simulink model "Test_FourMotor_PID_Ave"  (R2025a)
settings: Solver=ode4  StartTime=0.0  StopTime=2  FixedStep=60e-6  RelTol=1e-3
values from neighbouring files (symbols this model uses):
  Ts = 2e-6    (= 2e-06)    [param.m]
  ts_vec = 60e-6    (= 6e-05)    [param.m]
undefined symbols (not defined in the file or in its folder): DiscIntNeverNeededParam, gcbh, HEV_Param, Limit, magnitude, motorctrl, RPM, sps_rtmsupport
libraries: fl_lib x39, spsCurrentMeasurementLib x26, spsIdealSwitchLib x24, nesl_utility x22, spsVoltageMeasurementLib x21, simulink_extras x13, spsControlledCurrentSourceLib x12, spsControlledVoltageSourceLib x9, slpidlib x7, simulink x6, Uav_Electrical_lib x5, spsSeriesRLCBranchLib x4
(part 1 of 5)
settings Model: Creator=froshoo  LastModifiedBy=froshoo
settings DataIOCC: SaveOutput=off  SignalLogging=off  DSMLogging=off  SaveTime=off  ReturnWorkspaceOutputs=off
settings SimscapeCC: SimscapeLogType=all  SimscapeLogSimulationStatistics=on  SimscapeLogToSDI=on  SimscapeLogOpenViewer=on

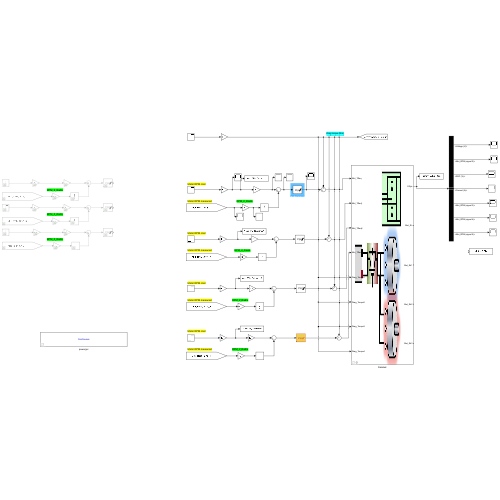
[thumbnail: Simulink's stored preview of the top-level diagram]
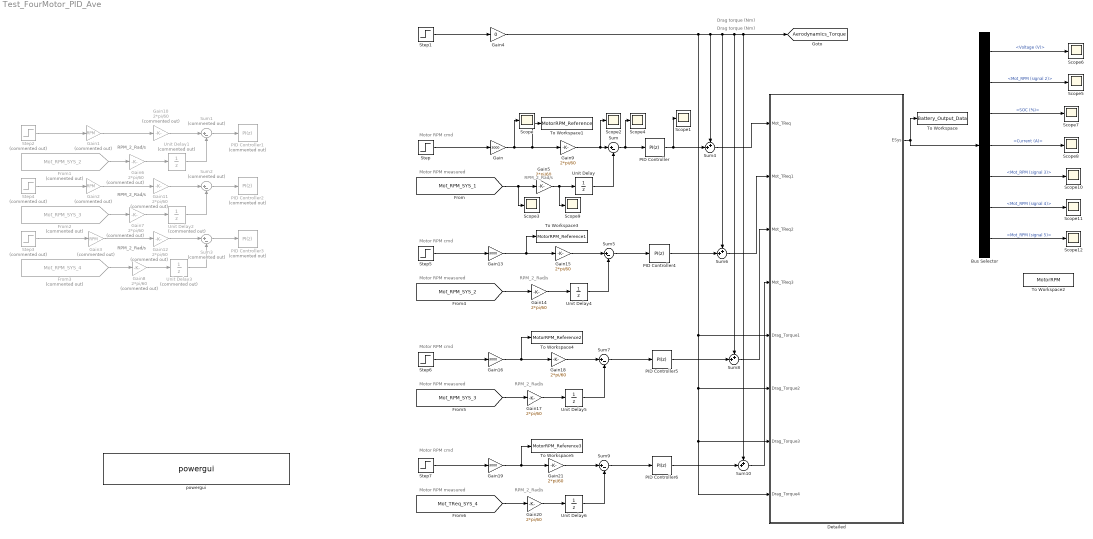
== system Test_FourMotor_PID_Ave ==
  note: Motor RPM cmd
  note: Motor RPM measured
  note: RPM_2_Rad/s
  note: RPM_2_Rad/s
  note: RPM_2_Rad/s
  note: RPM_2_Rad/s
  note: Drag torque (Nm)
  note: Drag torque (Nm)
  note: RPM_2_Rad/s
  note: Motor RPM cmd
  note: Motor RPM measured
  note: Motor RPM measured
  note: RPM_2_Rad/s
  note: Motor RPM cmd
  note: Motor RPM cmd
  note: Motor RPM measured
  note: RPM_2_Rad/s
  Bus Selector : BusSelector  OutputSignals=Batt (signal 1).Voltage (V),Mot_RPM (signal 2),Batt (signal 1).SOC (%),Batt (signal 1).Current (A),Mot_RPM (signal 3),Mot_RPM (signal 4),Mot_RPM (signal 5)
  Detailed : Subsystem  AncestorBlock=Uav_Electrical_lib/Detailed  mask{popup_batteryvariant=Cells}
      mask prompts: popup_batteryvariant "Battery Model"
      mask init:
      | set_param([gcb '/Battery'],'LabelModeActiveChoice',get_param(gcb,'popup_batteryvariant'));
      mask TypeOptions popup_batteryvariant: Predefined | Cells | Generic
      mask Display: image('HEV_Electrical_Detailed_IMAGE.jpg');
  From1 : From  Commented=on  GotoTag=Mot_RPM_SYS_2  TagVisibility=global
  From2 : From  Commented=on  GotoTag=Mot_RPM_SYS_3  TagVisibility=global
  From3 : From  Commented=on  GotoTag=Mot_RPM_SYS_4  TagVisibility=global
  Gain{,13,16,19} (4 alike) : Gain  Gain=3000
  Gain1 : Gain  Commented=on  Gain=RPM
  Gain{6..8,10..12} (6 alike) : Gain  Commented=on  Gain=2*pi/60
  Gain{5,9,14..15,17..18,20..21} (8 alike) : Gain  Gain=2*pi/60
  Gain2 : Gain  Commented=on  Gain=RPM
  Gain3 : Gain  Commented=on  Gain=RPM
  Gain4 : Gain  Gain=0
  PID Controller{,4..6} (4 alike) : slpidlib/PID Controller  Controller=PI  Form=Parallel  TimeDomain=Discrete-time  UseExternalTs=off  SampleTime=0.005  IntegratorMethod=Forward Euler  FilterMethod=Forward Euler  ControllerParametersSource=internal  P=0.4  I=0.5  UseKiTs=off  D=motorctrl.d  UseExternalDerivativeSource=off  N=motorctrl.n  UseFilter=on  TunerSelectOption=Transfer Function Based (PID Tuner App)  InitialConditionSource=internal  InitialConditionForIntegrator=0  InitialConditionForFilter=0  DifferentiatorICPrevScaledInput=0  ExternalReset=none  TrackingMode=off  Kt=1  LimitOutput=on  SatLimitsSource=internal  UpperSaturationLimit=800  LowerSaturationLimit=-800  LinearizeAsGain=on  AntiWindupMode=back-calculation  Kb=1  LimitIntegrator=off  UpperIntegratorSaturationLimit=inf  LowerIntegratorSaturationLimit=-inf  POutMin=[]  POutMax=[]  IOutMin=[]  IOutMax=[]  DOutMin=[]  DOutMax=[]  NOutMin=[]  NOutMax=[]  SumOutMin=[]  SumOutMax=[]  SaturationOutMin=[]  SaturationOutMax=[]  PParamMin=[]  PParamMax=[]  IParamMin=[]  IParamMax=[]  DParamMin=[]  DParamMax=[]  NParamMin=[]  NParamMax=[]  KbParamMin=[]  KbParamMax=[]  KtParamMin=[]  KtParamMax=[]  KbOutMin=[]  KbOutMax=[]  KtOutMin=[]  KtOutMax=[]  IntegratorOutMin=[]  IntegratorOutMax=[]  FilterOutMin=[]  FilterOutMax=[]  SumI1OutMin=[]  SumI1OutMax=[]  SumI2OutMin=[]  SumI2OutMax=[]  SumI3OutMin=[]  SumI3OutMax=[]  SumI4OutMin=[]  SumI4OutMax=[]  SumDOutMin=[]  SumDOutMax=[]  DifferentiatorOutMin=[]  DifferentiatorOutMax=[]  FilterDiffOutCoefMin=[]  FilterDiffOutCoefMax=[]  ReciprocalOutMin=[]  ReciprocalOutMax=[]  SumDenOutMin=[]  SumDenOutMax=[]  SumNumOutMin=[]  SumNumOutMax=[]  DivideOutMin=[]  DivideOutMax=[]  UdiffTsProdOutMin=[]  UdiffTsProdOutMax=[]  NTsProdOutMin=[]  NTsProdOutMax=[]  UintegralTsProdOutMin=[]  UintegralTsProdOutMax=[]  UngainTsProdOutMin=[]  UngainTsProdOutMax=[]  ClampingZeroOutDataTypeStr=Inherit: Inherit via back propagation  ClampingZeroOutMin=[]  ClampingZeroOutMax=[]  FilterDenConstantOutDataTypeStr=Inherit: Inherit via back propagation  FilterDenConstantOutMin=[]  FilterDenConstantOutMax=[]  PCopyOutDataTypeStr=Inherit: Inherit via back propagation  PCopyOutMin=[]  PCopyOutMax=[]  NCopyOutDataTypeStr=Inherit: Inherit via back propagation  NCopyOutMin=[]  NCopyOutMax=[]  IntegratorContinuousStateAttributes=''  IntegratorStateMustResolveToSignalObject=off  IntegratorRTWStateStorageClass=Auto  FilterContinuousStateAttributes=''  FilterStateMustResolveToSignalObject=off  FilterRTWStateStorageClass=Auto  ParallelPVariant=InternalParameters  IdealPVariant=Disabled  IVariant=InternalParameters  DVariant=Disabled  IntegratorVariant=Discrete  SatVariant=Enabled  AWVariant=BackCalculation  PCopyVariant=Disabled  TRVariant=Disabled  FdbkBlocksVariant=Forward  IdealPFdbkVariant=Disabled  SatFdbkVariant=Disabled  DerivativeFilterVariant=Disabled  NVariant=Disabled  NCopyVariant=Disabled_SignalSpec  FilterICVariant=Disabled  IntegratorICVariant=InternalICs  ExternalResetVariant=Disabled  TRSumVariant=Passthrough  SumFdbkVariant=Disabled  SumVariant=Sum_PI  TsampFilterVariant=InternalTs  TsampNgainVariant=Passthrough  TsampIntegralVariant=Disabled_SignalSpec  ExternalSaturationOutDataTypeStr=Inherit: Same as second input  DerivativeSourceVariant=Disabled  PreIntVariant=InternalPreInt
  PID Controller1 : slpidlib/PID Controller  Commented=on  Controller=PI  Form=Parallel  TimeDomain=Discrete-time  UseExternalTs=off  SampleTime=0.005  IntegratorMethod=Forward Euler  FilterMethod=Forward Euler  ControllerParametersSource=internal  P=motorctrl.p  I=motorctrl.i  UseKiTs=off  D=motorctrl.d  UseExternalDerivativeSource=off  N=motorctrl.n  UseFilter=on  TunerSelectOption=Transfer Function Based (PID Tuner App)  InitialConditionSource=internal  InitialConditionForIntegrator=0  InitialConditionForFilter=0  DifferentiatorICPrevScaledInput=0  ExternalReset=none  TrackingMode=off  Kt=1  LimitOutput=on  SatLimitsSource=internal  UpperSaturationLimit=Limit  LowerSaturationLimit=-Limit  LinearizeAsGain=on  AntiWindupMode=back-calculation  Kb=1  LimitIntegrator=off  UpperIntegratorSaturationLimit=inf  LowerIntegratorSaturationLimit=-inf  POutMin=[]  POutMax=[]  IOutMin=[]  IOutMax=[]  DOutMin=[]  DOutMax=[]  NOutMin=[]  NOutMax=[]  SumOutMin=[]  SumOutMax=[]  SaturationOutMin=[]  SaturationOutMax=[]  PParamMin=[]  PParamMax=[]  IParamMin=[]  IParamMax=[]  DParamMin=[]  DParamMax=[]  NParamMin=[]  NParamMax=[]  KbParamMin=[]  KbParamMax=[]  KtParamMin=[]  KtParamMax=[]  KbOutMin=[]  KbOutMax=[]  KtOutMin=[]  KtOutMax=[]  IntegratorOutMin=[]  IntegratorOutMax=[]  FilterOutMin=[]  FilterOutMax=[]  SumI1OutMin=[]  SumI1OutMax=[]  SumI2OutMin=[]  SumI2OutMax=[]  SumI3OutMin=[]  SumI3OutMax=[]  SumI4OutMin=[]  SumI4OutMax=[]  SumDOutMin=[]  SumDOutMax=[]  DifferentiatorOutMin=[]  DifferentiatorOutMax=[]  FilterDiffOutCoefMin=[]  FilterDiffOutCoefMax=[]  ReciprocalOutMin=[]  ReciprocalOutMax=[]  SumDenOutMin=[]  SumDenOutMax=[]  SumNumOutMin=[]  SumNumOutMax=[]  DivideOutMin=[]  DivideOutMax=[]  UdiffTsProdOutMin=[]  UdiffTsProdOutMax=[]  NTsProdOutMin=[]  NTsProdOutMax=[]  UintegralTsProdOutMin=[]  UintegralTsProdOutMax=[]  UngainTsProdOutMin=[]  UngainTsProdOutMax=[]  ClampingZeroOutDataTypeStr=Inherit: Inherit via back propagation  ClampingZeroOutMin=[]  ClampingZeroOutMax=[]  FilterDenConstantOutDataTypeStr=Inherit: Inherit via back propagation  FilterDenConstantOutMin=[]  FilterDenConstantOutMax=[]  PCopyOutDataTypeStr=Inherit: Inherit via back propagation  PCopyOutMin=[]  PCopyOutMax=[]  NCopyOutDataTypeStr=Inherit: Inherit via back propagation  NCopyOutMin=[]  NCopyOutMax=[]  IntegratorContinuousStateAttributes=''  IntegratorStateMustResolveToSignalObject=off  IntegratorRTWStateStorageClass=Auto  FilterContinuousStateAttributes=''  FilterStateMustResolveToSignalObject=off  FilterRTWStateStorageClass=Auto  ParallelPVariant=InternalParameters  IdealPVariant=Disabled  IVariant=InternalParameters  DVariant=Disabled  IntegratorVariant=Discrete  SatVariant=Enabled  AWVariant=BackCalculation  PCopyVariant=Disabled  TRVariant=Disabled  FdbkBlocksVariant=Forward  IdealPFdbkVariant=Disabled  SatFdbkVariant=Disabled  DerivativeFilterVariant=Disabled  NVariant=Disabled  NCopyVariant=Disabled_SignalSpec  FilterICVariant=Disabled  IntegratorICVariant=InternalICs  ExternalResetVariant=Disabled  TRSumVariant=Passthrough  SumFdbkVariant=Disabled  SumVariant=Sum_PI  TsampFilterVariant=InternalTs  TsampNgainVariant=Passthrough  TsampIntegralVariant=Disabled_SignalSpec  ExternalSaturationOutDataTypeStr=Inherit: Same as second input  DerivativeSourceVariant=Disabled  PreIntVariant=InternalPreInt
  PID Controller2 : slpidlib/PID Controller  Commented=on  Controller=PI  Form=Parallel  TimeDomain=Discrete-time  UseExternalTs=off  SampleTime=0.005  IntegratorMethod=Forward Euler  FilterMethod=Forward Euler  ControllerParametersSource=internal  P=motorctrl.p  I=motorctrl.i  UseKiTs=off  D=motorctrl.d  UseExternalDerivativeSource=off  N=motorctrl.n  UseFilter=on  TunerSelectOption=Transfer Function Based (PID Tuner App)  InitialConditionSource=internal  InitialConditionForIntegrator=0  InitialConditionForFilter=0  DifferentiatorICPrevScaledInput=0  ExternalReset=none  TrackingMode=off  Kt=1  LimitOutput=on  SatLimitsSource=internal  UpperSaturationLimit=Limit  LowerSaturationLimit=-Limit  LinearizeAsGain=on  AntiWindupMode=back-calculation  Kb=1  LimitIntegrator=off  UpperIntegratorSaturationLimit=inf  LowerIntegratorSaturationLimit=-inf  POutMin=[]  POutMax=[]  IOutMin=[]  IOutMax=[]  DOutMin=[]  DOutMax=[]  NOutMin=[]  NOutMax=[]  SumOutMin=[]  SumOutMax=[]  SaturationOutMin=[]  SaturationOutMax=[]  PParamMin=[]  PParamMax=[]  IParamMin=[]  IParamMax=[]  DParamMin=[]  DParamMax=[]  NParamMin=[]  NParamMax=[]  KbParamMin=[]  KbParamMax=[]  KtParamMin=[]  KtParamMax=[]  KbOutMin=[]  KbOutMax=[]  KtOutMin=[]  KtOutMax=[]  IntegratorOutMin=[]  IntegratorOutMax=[]  FilterOutMin=[]  FilterOutMax=[]  SumI1OutMin=[]  SumI1OutMax=[]  SumI2OutMin=[]  SumI2OutMax=[]  SumI3OutMin=[]  SumI3OutMax=[]  SumI4OutMin=[]  SumI4OutMax=[]  SumDOutMin=[]  SumDOutMax=[]  DifferentiatorOutMin=[]  DifferentiatorOutMax=[]  FilterDiffOutCoefMin=[]  FilterDiffOutCoefMax=[]  ReciprocalOutMin=[]  ReciprocalOutMax=[]  SumDenOutMin=[]  SumDenOutMax=[]  SumNumOutMin=[]  SumNumOutMax=[]  DivideOutMin=[]  DivideOutMax=[]  UdiffTsProdOutMin=[]  UdiffTsProdOutMax=[]  NTsProdOutMin=[]  NTsProdOutMax=[]  UintegralTsProdOutMin=[]  UintegralTsProdOutMax=[]  UngainTsProdOutMin=[]  UngainTsProdOutMax=[]  ClampingZeroOutDataTypeStr=Inherit: Inherit via back propagation  ClampingZeroOutMin=[]  ClampingZeroOutMax=[]  FilterDenConstantOutDataTypeStr=Inherit: Inherit via back propagation  FilterDenConstantOutMin=[]  FilterDenConstantOutMax=[]  PCopyOutDataTypeStr=Inherit: Inherit via back propagation  PCopyOutMin=[]  PCopyOutMax=[]  NCopyOutDataTypeStr=Inherit: Inherit via back propagation  NCopyOutMin=[]  NCopyOutMax=[]  IntegratorContinuousStateAttributes=''  IntegratorStateMustResolveToSignalObject=off  IntegratorRTWStateStorageClass=Auto  FilterContinuousStateAttributes=''  FilterStateMustResolveToSignalObject=off  FilterRTWStateStorageClass=Auto  ParallelPVariant=InternalParameters  IdealPVariant=Disabled  IVariant=InternalParameters  DVariant=Disabled  IntegratorVariant=Discrete  SatVariant=Enabled  AWVariant=BackCalculation  PCopyVariant=Disabled  TRVariant=Disabled  FdbkBlocksVariant=Forward  IdealPFdbkVariant=Disabled  SatFdbkVariant=Disabled  DerivativeFilterVariant=Disabled  NVariant=Disabled  NCopyVariant=Disabled_SignalSpec  FilterICVariant=Disabled  IntegratorICVariant=InternalICs  ExternalResetVariant=Disabled  TRSumVariant=Passthrough  SumFdbkVariant=Disabled  SumVariant=Sum_PI  TsampFilterVariant=InternalTs  TsampNgainVariant=Passthrough  TsampIntegralVariant=Disabled_SignalSpec  ExternalSaturationOutDataTypeStr=Inherit: Same as second input  DerivativeSourceVariant=Disabled  PreIntVariant=InternalPreInt
  PID Controller3 : slpidlib/PID Controller  Commented=on  Controller=PI  Form=Parallel  TimeDomain=Discrete-time  UseExternalTs=off  SampleTime=0.005  IntegratorMethod=Forward Euler  FilterMethod=Forward Euler  ControllerParametersSource=internal  P=motorctrl.p  I=motorctrl.i  UseKiTs=off  D=motorctrl.d  UseExternalDerivativeSource=off  N=motorctrl.n  UseFilter=on  TunerSelectOption=Transfer Function Based (PID Tuner App)  InitialConditionSource=internal  InitialConditionForIntegrator=0  InitialConditionForFilter=0  DifferentiatorICPrevScaledInput=0  ExternalReset=none  TrackingMode=off  Kt=1  LimitOutput=on  SatLimitsSource=internal  UpperSaturationLimit=Limit  LowerSaturationLimit=-Limit  LinearizeAsGain=on  AntiWindupMode=back-calculation  Kb=1  LimitIntegrator=off  UpperIntegratorSaturationLimit=inf  LowerIntegratorSaturationLimit=-inf  POutMin=[]  POutMax=[]  IOutMin=[]  IOutMax=[]  DOutMin=[]  DOutMax=[]  NOutMin=[]  NOutMax=[]  SumOutMin=[]  SumOutMax=[]  SaturationOutMin=[]  SaturationOutMax=[]  PParamMin=[]  PParamMax=[]  IParamMin=[]  IParamMax=[]  DParamMin=[]  DParamMax=[]  NParamMin=[]  NParamMax=[]  KbParamMin=[]  KbParamMax=[]  KtParamMin=[]  KtParamMax=[]  KbOutMin=[]  KbOutMax=[]  KtOutMin=[]  KtOutMax=[]  IntegratorOutMin=[]  IntegratorOutMax=[]  FilterOutMin=[]  FilterOutMax=[]  SumI1OutMin=[]  SumI1OutMax=[]  SumI2OutMin=[]  SumI2OutMax=[]  SumI3OutMin=[]  SumI3OutMax=[]  SumI4OutMin=[]  SumI4OutMax=[]  SumDOutMin=[]  SumDOutMax=[]  DifferentiatorOutMin=[]  DifferentiatorOutMax=[]  FilterDiffOutCoefMin=[]  FilterDiffOutCoefMax=[]  ReciprocalOutMin=[]  ReciprocalOutMax=[]  SumDenOutMin=[]  SumDenOutMax=[]  SumNumOutMin=[]  SumNumOutMax=[]  DivideOutMin=[]  DivideOutMax=[]  UdiffTsProdOutMin=[]  UdiffTsProdOutMax=[]  NTsProdOutMin=[]  NTsProdOutMax=[]  UintegralTsProdOutMin=[]  UintegralTsProdOutMax=[]  UngainTsProdOutMin=[]  UngainTsProdOutMax=[]  ClampingZeroOutDataTypeStr=Inherit: Inherit via back propagation  ClampingZeroOutMin=[]  ClampingZeroOutMax=[]  FilterDenConstantOutDataTypeStr=Inherit: Inherit via back propagation  FilterDenConstantOutMin=[]  FilterDenConstantOutMax=[]  PCopyOutDataTypeStr=Inherit: Inherit via back propagation  PCopyOutMin=[]  PCopyOutMax=[]  NCopyOutDataTypeStr=Inherit: Inherit via back propagation  NCopyOutMin=[]  NCopyOutMax=[]  IntegratorContinuousStateAttributes=''  IntegratorStateMustResolveToSignalObject=off  IntegratorRTWStateStorageClass=Auto  FilterContinuousStateAttributes=''  FilterStateMustResolveToSignalObject=off  FilterRTWStateStorageClass=Auto  ParallelPVariant=InternalParameters  IdealPVariant=Disabled  IVariant=InternalParameters  DVariant=Disabled  IntegratorVariant=Discrete  SatVariant=Enabled  AWVariant=BackCalculation  PCopyVariant=Disabled  TRVariant=Disabled  FdbkBlocksVariant=Forward  IdealPFdbkVariant=Disabled  SatFdbkVariant=Disabled  DerivativeFilterVariant=Disabled  NVariant=Disabled  NCopyVariant=Disabled_SignalSpec  FilterICVariant=Disabled  IntegratorICVariant=InternalICs  ExternalResetVariant=Disabled  TRSumVariant=Passthrough  SumFdbkVariant=Disabled  SumVariant=Sum_PI  TsampFilterVariant=InternalTs  TsampNgainVariant=Passthrough  TsampIntegralVariant=Disabled_SignalSpec  ExternalSaturationOutDataTypeStr=Inherit: Same as second input  DerivativeSourceVariant=Disabled  PreIntVariant=InternalPreInt
  Scope{,1..12} (13 alike) : Scope
      Scope settings: ActiveDisplayYMinimum=2000  ActiveDisplayYMaximum=4000
      Scope1 settings: ActiveDisplayYMinimum=-481.89960137193771  ActiveDisplayYMaximum=332.79708047153025
      Scope10 settings: ActiveDisplayYMinimum=-838.99189969639019  ActiveDisplayYMaximum=7550.927097267514  DataLoggingVariableName=ScopeData18
      Scope11 settings: ActiveDisplayYMinimum=-838.99189969639019  ActiveDisplayYMaximum=7550.927097267514  DataLoggingVariableName=ScopeData22
      Scope12 settings: ActiveDisplayYMinimum=-838.99189969639019  ActiveDisplayYMaximum=7550.927097267514  DataLoggingVariableName=ScopeData23
      Scope2 settings: ActiveDisplayYMinimum=214.15926535897933  ActiveDisplayYMaximum=414.15926535897933  DataLoggingVariableName=ScopeData17
      Scope3 settings: ActiveDisplayYMinimum=-1  ActiveDisplayYMaximum=1  DataLoggingVariableName=ScopeData19
      Scope4 settings: ActiveDisplayYMinimum=-39.421537573321494  ActiveDisplayYMaximum=353.44602124034606  DataLoggingVariableName=ScopeData20
      Scope5 settings: ActiveDisplayYMinimum=-838.99189969639019  ActiveDisplayYMaximum=7550.927097267514  DataLoggingVariableName=ScopeData2
      Scope6 settings: ActiveDisplayYMinimum=813.40102643578655  ActiveDisplayYMaximum=813.74696487540177  DataLoggingVariableName=ScopeData3
      Scope7 settings: ActiveDisplayYMinimum=99.00226  ActiveDisplayYMaximum=100.11086  DataLoggingVariableName=ScopeData4
      Scope8 settings: ActiveDisplayYMinimum=-1508.9225284750978  ActiveDisplayYMaximum=1817.2458957057474  DataLoggingVariableName=ScopeData5
      Scope9 settings: ActiveDisplayYMinimum=-39.286755881366751  ActiveDisplayYMaximum=353.5808029323008  DataLoggingVariableName=ScopeData21
  Step{,1,5..7} (5 alike) : Step  Time=0  SampleTime=0
  Step2 : Step  Commented=on  Time=0  SampleTime=0
  Step3 : Step  Commented=on  Time=0  SampleTime=0
  Step4 : Step  Commented=on  Time=0  SampleTime=0
  Sum{,5,7,9} (4 alike) : Sum  Inputs=|+-
  Sum1 : Sum  Commented=on  Inputs=|+-
  Sum{4,6,8,10} (4 alike) : Sum  Inputs=++|
  Sum2 : Sum  Commented=on  Inputs=|+-
  Sum3 : Sum  Commented=on  Inputs=|+-
  To Workspace : ToWorkspace  VariableName=Battery_Output_Data  SaveFormat=Timeseries  SampleTime=-1
  To Workspace1 : ToWorkspace  VariableName=MotorRPM_Reference  SaveFormat=Timeseries  SampleTime=-1
  To Workspace2 : ToWorkspace  VariableName=MotorRPM  SaveFormat=Timeseries  SampleTime=-1
  To Workspace3 : ToWorkspace  VariableName=MotorRPM_Reference1  SaveFormat=Timeseries  SampleTime=-1
  To Workspace4 : ToWorkspace  VariableName=MotorRPM_Reference2  SaveFormat=Timeseries  SampleTime=-1
  To Workspace5 : ToWorkspace  VariableName=MotorRPM_Reference3  SaveFormat=Timeseries  SampleTime=-1
  Unit Delay{,4..6} (4 alike) : UnitDelay  SampleTime=-1  HasFrameUpgradeWarning=on
  Unit Delay1 : UnitDelay  Commented=on  SampleTime=-1  HasFrameUpgradeWarning=on
  Unit Delay2 : UnitDelay  Commented=on  SampleTime=-1  HasFrameUpgradeWarning=on
  Unit Delay3 : UnitDelay  Commented=on  SampleTime=-1  HasFrameUpgradeWarning=on
  powergui : sps_lib/powergui  Priority=1  SimulationMode=Continuous  SampleTime=50e-6  frequency=60  Iterations=50  frequencyindice=0  Pbase=100e6  ErrMax=1e-4  UnitsV=kV  UnitsW=MW  buscounter=0  FunctionMessages=off  echomessages=off  EnableUseOfTLC=off  CurrentSourceSwitches=off  DisableSnubberDevices=off  DisableRonSwitches=off  DisableVfSwitches=off  DisplayEquations=off  AutomaticDiscreteSolvers=off  SolverType=Tustin/Backward Euler (TBE)  Interpol=off  ExternalGateDelay=off  methode=off  Ts=100  x0status=blocks  SPID=on  SwTol=0  HookPort=off  NonlinearTolerance=1e-4  nMaxIteration=100  ContinueOnMaxIteration=off  RestoreLinks=warning  ResistiveCurrentMeasurement=off  Frange=[0:2:500]  Ylog=off  Xlog=on  ShowGrid=off  save=off  variable=ZData  structure=0  ZoomFFT=off  StartTime=0.0  cycles=1  DisplayStyle=1  fundamental=60  FreqAxis=off  MaxFrequency=1000  frequencyindicesteady=1  RmsSteady=1  display=off
  tag scope: Aerodynamics_Torque=global
  wires:
  Sum/1 -> Scope4/1, PID Controller/1
  From1/1 -> Gain6/1
  Sum1/1 -> PID Controller1/1
  Sum2/1 -> PID Controller2/1
  From3/1 -> Gain8/1
  Sum3/1 -> PID Controller3/1
  Detailed/1(ESys) -> To Workspace/1, Bus Selector/1
  Step/1 -> Gain/1
  Step3/1 -> Gain3/1
  Step4/1 -> Gain2/1
  Step2/1 -> Gain1/1
  Gain/1 -> To Workspace1/1, Gain9/1, Scope/1
  Gain1/1 -> Gain10/1
  Gain2/1 -> Gain11/1
  Gain3/1 -> Gain12/1
  [Mot_RPM_SYS_1] -> Gain5/1, Scope3/1
  Unit Delay/1 -> Sum/2
  Unit Delay1/1 -> Sum1/2
  Unit Delay2/1 -> Sum2/2
  Unit Delay3/1 -> Sum3/2
  From2/1 -> Gain7/1
  Step1/1 -> Gain4/1
  Gain5/1 -> Scope9/1, Unit Delay/1
  Gain6/1 -> Unit Delay1/1
  Gain7/1 -> Unit Delay2/1
  Gain8/1 -> Unit Delay3/1
  Gain9/1 -> Scope2/1, Sum/1
  Gain10/1 -> Sum1/1
  Gain11/1 -> Sum2/1
  Gain12/1 -> Sum3/1
  PID Controller/1 -> Sum4/2, Scope1/1
  Sum4/1 -> Detailed/1(Mot_TReq)
  PID Controller4/1 -> Sum6/2
  Gain15/1 -> Sum5/1
  Sum5/1 -> PID Controller4/1
  [Mot_RPM_SYS_2] -> Gain14/1
  Sum6/1 -> Detailed/2(Mot_TReq1)
  Step5/1 -> Gain13/1
  Gain14/1 -> Unit Delay4/1
  Unit Delay4/1 -> Sum5/2
  Gain13/1 -> To Workspace3/1, Gain15/1
  Sum7/1 -> PID Controller5/1
  Gain18/1 -> Sum7/1
  PID Controller5/1 -> Sum8/2
  Gain17/1 -> Unit Delay5/1
  Step6/1 -> Gain16/1
  Gain16/1 -> To Workspace4/1, Gain18/1
  Sum8/1 -> Detailed/3(Mot_TReq2)
  [Mot_RPM_SYS_3] -> Gain17/1
  Unit Delay5/1 -> Sum7/2
  Unit Delay6/1 -> Sum9/2
  Gain21/1 -> Sum9/1
  Sum10/1 -> Detailed/4(Mot_TReq3)
  Step7/1 -> Gain19/1
  PID Controller6/1 -> Sum10/2
  Sum9/1 -> PID Controller6/1
  Gain19/1 -> To Workspace5/1, Gain21/1
  Gain20/1 -> Unit Delay6/1
  [Mot_TReq_SYS_4] -> Gain20/1
  Gain4/1 -> Detailed/5(Drag_Torque1), Detailed/6(Drag_Torque2), Detailed/7(Drag_Torque3), Detailed/8(Drag_Torque4), [Aerodynamics_Torque], Sum10/1, Sum8/1, Sum6/1, Sum4/1
  Bus Selector/1 -> Scope6/1  "<Voltage (V)>"
  Bus Selector/2 -> Scope5/1  "<Mot_RPM (signal 2)>"
  Bus Selector/3 -> Scope7/1  "<SOC (%)>"
  Bus Selector/4 -> Scope8/1  "<Current (A)>"
  Bus Selector/5 -> Scope10/1  "<Mot_RPM (signal 3)>"
  Bus Selector/6 -> Scope11/1  "<Mot_RPM (signal 4)>"
  Bus Selector/7 -> Scope12/1  "<Mot_RPM (signal 5)>"

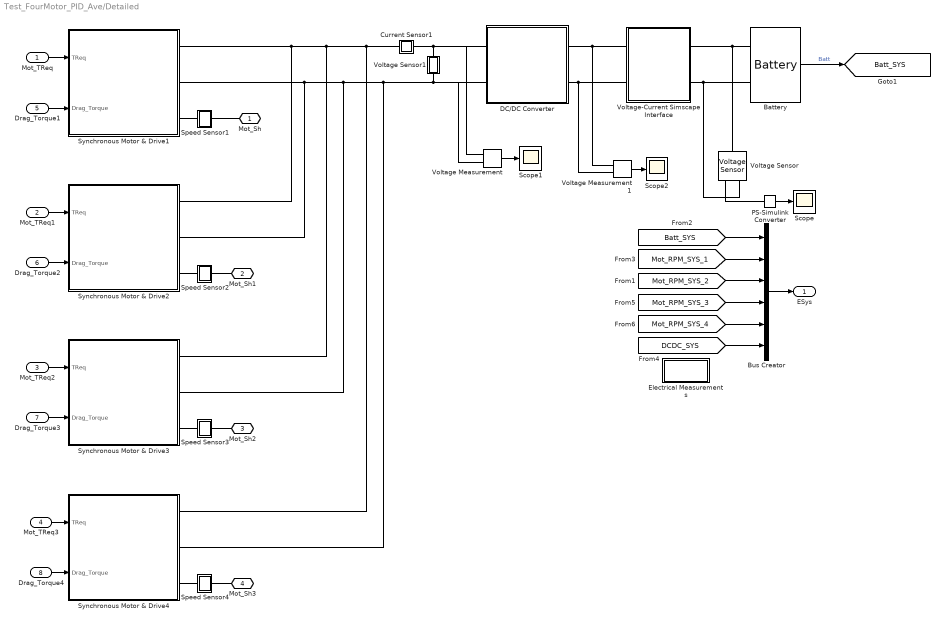
== system Test_FourMotor_PID_Ave/Detailed ==
  Mot_TReq : Inport
  Mot_TReq1 : Inport  Port=2
  Mot_TReq2 : Inport  Port=3
  Mot_TReq3 : Inport  Port=4
  Drag_Torque1 : Inport  Port=5
  Drag_Torque2 : Inport  Port=6
  Drag_Torque3 : Inport  Port=7
  Drag_Torque4 : Inport  Port=8
  Battery : HEV_Battery_Lib/Battery  SystemSampleTime=-1  LabelModeActiveChoice=Cells  VariantActivationTime=update diagram  EmptyChoice=off  PassThrough=off  PassThroughVariantControl=(default)  EmptyChoiceVariantControl=(default)  AllowFlexibleInterface=on  Latency=0  AutoFrameSizeCalculation=off
  Bus Creator : BusCreator  Inputs=6
  Current Sensor1 : Subsystem
  DC/DC Converter : Subsystem
      mask Display:
      | image(imread('HEV_DCDC_Switching_IMAGE.jpg'));
      | port_label('RConn',1,'Bus+');
      | port_label('RConn',2,'Bus-');
      | port_label('LConn',1,'Batt+');
      | port_label('LConn',2,'Batt-');
      | text(0.05,0.5,'Out');
      | text(0.85,0.5,'In');
  Electrical Measurements : Subsystem
  PS-Simulink Converter : nesl_utility/PS-Simulink Converter  PhysicalDomain=network_engine_domain  SubClassName=ps_output  LeftPortType=input  RightPortType=output  PseudoPeriodic=off  Frequencies=[]  VectorFormat=inherit  Unit=inherit  AffineConversion=off
  Scope : Scope
      settings: ActiveDisplayYMinimum=-36.23924195513996  ActiveDisplayYMaximum=868.21914969835188  DataLoggingVariableName=ScopeData8
  Scope1 : Scope
      settings: ActiveDisplayYMinimum=153.22209455008215  ActiveDisplayYMaximum=2647.7003324838884  DataLoggingVariableName=ScopeData9
  Scope2 : Scope
      settings: ActiveDisplayYMinimum=-104.13434216137392  ActiveDisplayYMaximum=931.66530804851823  DataLoggingVariableName=ScopeData10
  Speed Sensor1 : Subsystem
      mask Display: disp('S');
  Speed Sensor2 : Subsystem
      mask Display: disp('S');
  Speed Sensor3 : Subsystem
      mask Display: disp('S');
  Speed Sensor4 : Subsystem
      mask Display: disp('S');
  Synchronous Motor & Drive1 : Subsystem
      mask Display:
      | image(imread('HEV_Detailed_Motor_IMAGE.jpg'));
      | port_label('input',1,'T_Req');
      | port_label('RConn',1,'+');
      | port_label('RConn',2,'-');
      | port_label('RConn',3,'Shaft');
  Synchronous Motor & Drive2 : Subsystem
      mask Display:
      | image(imread('HEV_Detailed_Motor_IMAGE.jpg'));
      | port_label('input',1,'T_Req');
      | port_label('RConn',1,'+');
      | port_label('RConn',2,'-');
      | port_label('RConn',3,'Shaft');
  Synchronous Motor & Drive3 : Subsystem
      mask Display:
      | image(imread('HEV_Detailed_Motor_IMAGE.jpg'));
      | port_label('input',1,'T_Req');
      | port_label('RConn',1,'+');
      | port_label('RConn',2,'-');
      | port_label('RConn',3,'Shaft');
  Synchronous Motor & Drive4 : Subsystem
      mask Display:
      | image(imread('HEV_Detailed_Motor_IMAGE.jpg'));
      | port_label('input',1,'T_Req');
      | port_label('RConn',1,'+');
      | port_label('RConn',2,'-');
      | port_label('RConn',3,'Shaft');
  Voltage Sensor1 : Subsystem
  Voltage Measurement : spsVoltageMeasurementLib/Voltage Measurement  PhasorSimulation=off  OutputType=Complex  PSBequivalent=0
  Voltage Measurement1 : spsVoltageMeasurementLib/Voltage Measurement  PhasorSimulation=off  OutputType=Complex  PSBequivalent=0
  Voltage Sensor : fl_lib/Electrical/Electrical Sensors/Voltage Sensor
  Voltage-Current Simscape Interface : Subsystem  AncestorBlock=sps_lib/Utilities/Voltage-Current Simscape Interface  LoadFcn=sps_rtmsupport('LoadFcn',gcbh);  StartFcn=sps_rtmsupport('StartFcn',gcbh);  StopFcn=sps_rtmsupport('StopFcn',gcbh);  mask(Specialized Power Systems - Simscape Interface Element){DFT=off, Fmode=Low pass filter (continuous), T=1e-6, Ts=50e-6, i0=0, v0=0, Sd=Specialized Power Systems side, Measurements=off}
      mask prompts: DFT "Direct feedthrough (no filter)"; Fmode "Filter type:"; T "Low pass filter time constant (s):"; Ts "Sample time (s):"; i0 "Initial current (A):"; v0 "Initial voltage (V):"; Sd "Apply filter on:"; Measurements "Show measurement ports"
      mask help:
      | Represents an ideal coupling between Specialized Power Systems and Simscape circuit.
      |
      | The block acts as a voltage source on the Specialized Power Systems side, and as a current source on the Simscape side.
      |
      | The filter can be specified to break algebraic loop between Specialized Power Systems and Simscape circuits.
      mask init:
      | x0=0;%default value
      | [T_PS,x0] = powericon('InterfaceElementCback',gcb,'init',0,DFT,Fmode,T,Ts,i0,v0,Sd,Measurements);
      settings: CopyFcn=sps_rtmsupport('CopyFcn',gcbh);  DeleteFcn=sps_rtmsupport('DeleteFcn',gcbh);  UndoDeleteFcn=sps_rtmsupport('UndoDeleteFcn',gcbh);  ModelCloseFcn=sps_rtmsupport('ModelCloseFcn',gcbh);  PreSaveFcn=sps_rtmsupport('PreSaveFcn',gcbh);  PostSaveFcn=sps_rtmsupport('PostSaveFcn',gcbh);  NameChangeFcn=sps_rtmsupport('NameChangeFcn',gcbh);  PreCopyFcn=sps_rtmsupport('PreCopyFcn',gcbh);  OpenFcn=sps_rtmsupport('OpenFcn',gcbh, [1 2 7 8]);  CloseFcn=sps_rtmsupport('CloseFcn',gcbh);  PreDeleteFcn=sps_rtmsupport('PreDeleteFcn',gcbh);
      settings: LibrarySourceBlock=|
      | sps_lib/Utilities/Voltage-Current
      | Simscape Interface
      mask Help: helpview(psbhelp('Voltage-Current Simscape Interface'));
      mask Callback DFT: powericon('InterfaceElementCback',gcbh,'mask',0);
      mask TypeOptions Fmode: Low pass filter (continuous) | Unit delay (discrete) | First-order input filtering | Second-order input filtering
      mask Callback Fmode: powericon('InterfaceElementCback',gcbh,'mask',0);
      mask TypeOptions Sd: Specialized Power Systems side | Simscape side
      mask Callback Sd: powericon('InterfaceElementCback',gcbh,'mask',0);
      mask Display:
      | color('blue')
      | disp('V-I')
  Mot_Sh : PMIOPort  Side=Right
  Mot_Sh1 : PMIOPort  Port=2  Side=Right
  Mot_Sh2 : PMIOPort  Port=3  Side=Right
  Mot_Sh3 : PMIOPort  Port=4  Side=Right
  ESys : Outport  VectorParamsAs1DForOutWhenUnconnected=off
  tag scope: Batt_SYS=global
  wires:
  [Batt_SYS] -> Bus Creator/1
  Bus Creator/1 -> ESys/1
  Battery/1 -> [Batt_SYS]  "Batt"
  Mot_TReq/1 -> Synchronous Motor & Drive1/1(TReq)
  Voltage Measurement/1 -> Scope1/1
  Voltage Measurement1/1 -> Scope2/1
  [Mot_RPM_SYS_1] -> Bus Creator/2
  PS-Simulink Converter/1 -> Scope/1
  Mot_TReq1/1 -> Synchronous Motor & Drive2/1(TReq)
  Mot_TReq2/1 -> Synchronous Motor & Drive3/1(TReq)
  Mot_TReq3/1 -> Synchronous Motor & Drive4/1(TReq)
  Drag_Torque1/1 -> Synchronous Motor & Drive1/2(Drag_Torque)
  Drag_Torque4/1 -> Synchronous Motor & Drive4/2(Drag_Torque)
  Drag_Torque3/1 -> Synchronous Motor & Drive3/2(Drag_Torque)
  Drag_Torque2/1 -> Synchronous Motor & Drive2/2(Drag_Torque)
  [Mot_RPM_SYS_2] -> Bus Creator/3
  [Mot_RPM_SYS_3] -> Bus Creator/4
  [Mot_RPM_SYS_4] -> Bus Creator/5
  [DCDC_SYS] -> Bus Creator/6
  connections:
  Mot_Sh/RConn1 -- Speed Sensor1/RConn1
  Speed Sensor1/LConn1 -- Synchronous Motor & Drive1/RConn3
  Current Sensor1/LConn1 -- Synchronous Motor & Drive4/RConn1 -- Synchronous Motor & Drive3/RConn1 -- Synchronous Motor & Drive1/RConn1 -- Synchronous Motor & Drive2/RConn1
  Voltage Sensor1/RConn1 -- Voltage Measurement/LConn1 -- DC/DC Converter/RConn1 -- Current Sensor1/RConn1
  Battery/LConn2 -- Voltage Sensor/RConn2 -- Voltage-Current Simscape Interface/RConn2
  Voltage-Current Simscape Interface/LConn1 -- Voltage Measurement1/LConn1 -- DC/DC Converter/LConn1
  Voltage-Current Simscape Interface/LConn2 -- Voltage Measurement1/LConn2 -- DC/DC Converter/LConn2
  Voltage-Current Simscape Interface/RConn1 -- Battery/LConn1 -- Voltage Sensor/LConn1
  PS-Simulink Converter/LConn1 -- Voltage Sensor/RConn1
  Voltage Sensor1/LConn1 -- Synchronous Motor & Drive4/RConn2 -- Synchronous Motor & Drive3/RConn2 -- Synchronous Motor & Drive2/RConn2 -- Synchronous Motor & Drive1/RConn2 -- DC/DC Converter/RConn2 -- Voltage Measurement/LConn2
  Speed Sensor2/LConn1 -- Synchronous Motor & Drive2/RConn3
  Mot_Sh1/RConn1 -- Speed Sensor2/RConn1
  Speed Sensor3/LConn1 -- Synchronous Motor & Drive3/RConn3
  Mot_Sh2/RConn1 -- Speed Sensor3/RConn1
  Mot_Sh3/RConn1 -- Speed Sensor4/RConn1
  Speed Sensor4/LConn1 -- Synchronous Motor & Drive4/RConn3

== system Test_FourMotor_PID_Ave/Detailed/Current Sensor1 ==
  i1 : spsCurrentMeasurementLib/Current Measurement  PhasorSimulation=off  OutputType=Complex  PSBequivalent=0
  - : PMIOPort  Side=Left
  + : PMIOPort  Tag=PMCPort  Port=2  Side=Right
  tag scope: Mot_Current_SYS=global
  wires:
  i1/1 -> [Mot_Current_SYS]
  connections:
  -/RConn1 -- i1/RConn1
  +/RConn1 -- i1/LConn1

== system Test_FourMotor_PID_Ave/Detailed/DC//DC Converter ==
  CBus : spsSeriesRLCBranchLib/Series RLC Branch  LConnTagsString=__new0  RConnTagsString=__new0  BranchType=RC  Resistance=0.1  Inductance=1e-3  SetiL0=off  InitialCurrent=0  Capacitance=1130e-6  Setx0=on  InitialVoltage=800  Measurements=None
  CBus1 : spsSeriesRLCBranchLib/Series RLC Branch  LConnTagsString=__new0  RConnTagsString=__new0  BranchType=C  Resistance=0.2  Inductance=1e-3  SetiL0=off  InitialCurrent=0  Capacitance=282e-6  Setx0=on  InitialVoltage=150  Measurements=None
  Detailed Boost converter : spsUniversalBridgeLib/Universal Bridge  Arms=1  SnubberResistance=5000  SnubberCapacitance=inf  Device=IGBT / Diodes  Ron=1e-3  Lon=0  ForwardVoltages=[0,0]  ForwardVoltage=0  GTOparameters=[ 10e-6 , 20e-6 ]  IGBTparameters=[0,0]  Measurements=None  Measurements_2=None  converterType=Rectifier
  L : spsSeriesRLCBranchLib/Series RLC Branch  LConnTagsString=__new0  RConnTagsString=__new0  BranchType=L  Resistance=0.3  Inductance=373e-6  SetiL0=off  InitialCurrent=100  Capacitance=100e-6  Setx0=off  InitialVoltage=0  Measurements=None
  PWM : Subsystem
  Ubus Ref : Constant  Value=HEV_Param.DCDCConv.Output_Voltage
  V1 : spsVoltageMeasurementLib/Voltage Measurement  PhasorSimulation=off  OutputType=Complex  PSBequivalent=0
  Voltage Controller : Subsystem  mask(PI controller){Kp=0.001, Ki=1, Ts=0.002}
      mask prompts: Kp "Proportional gain (Kp)"; Ki "Integral gain (Ki)"; Ts "Sample time (s) :"
      mask help: Proportional-Integral Speed Controller
      mask Display: plot(0,0,100,100,[35,35,65],[70,30,30],[35,65],[45,60])
  Bus+ : PMIOPort  Tag=PMCPort  Side=Right
  Bus- : PMIOPort  Tag=PMCPort  Port=2  Side=Right
  Batt+ : PMIOPort  Tag=PMCPort  Port=3  Side=Left
  Batt- : PMIOPort  Tag=PMCPort  Port=4  Side=Left
  wires:
  PWM/1(Pulses) -> Detailed Boost converter/1
  Voltage Controller/1(Ec) -> PWM/1(Ref.)
  Ubus Ref/1 -> Voltage Controller/1(Uref)
  V1/1 -> Voltage Controller/2(UBus)
  connections:
  L/LConn1 -- Detailed Boost converter/LConn1
  Detailed Boost converter/RConn1 -- CBus/LConn1 -- V1/LConn1 -- Bus+/RConn1
  Batt+/RConn1 -- L/RConn1 -- CBus1/LConn1
  Detailed Boost converter/RConn2 -- CBus1/RConn1 -- Batt-/RConn1 -- Bus-/RConn1 -- CBus/RConn1 -- V1/LConn2

== system Test_FourMotor_PID_Ave/Detailed/Electrical Measurements ==
  Bus Selector : BusSelector  OutputSignals=Voltage (V),Current (A),SOC (%)
  Mux : Mux  Inputs=2
  Mux1 : Mux  Inputs=3
  Mux2 : Mux  Inputs=3
  Mux3 : Mux
  Mux4 : Mux  Inputs=2
  Product1 : Product  RndMeth=Zero
  Product2 : Product  RndMeth=Zero
  Product3 : Product  RndMeth=Zero
  tag scope: Electricals=global, Power=global
  wires:
  Product2/1 -> Mux1/1  "Motor Power (W)"
  Product1/1 -> Mux1/2  "Generator power (W)"
  Product3/1 -> Mux1/3  "Battery power (W)"
  [Mot_Current_SYS] -> Product2/1, Mux2/1
  Mux1/1 -> [Power]
  [Batt_Measures] -> Bus Selector/1
  Bus Selector/1 -> Mux/2, Product3/1  "<Voltage (V)>"
  Bus Selector/2 -> Product3/2, Mux2/2  "<Current (A)>"
  Mux/1 -> Mux3/2  "Voltage (DC bus, Battery)"
  Mux2/1 -> Mux3/3  "Current (Motor, Battery, Generator)"
  [Gen_Current_SYS] -> Product1/1, Mux2/3
  Bus Selector/3 -> Mux3/4  "<SOC (%)>"
  [DC_Bus_SYS] -> Product2/2, Product1/2, Mux/1, Mux4/1, Mux4/2
  Mux3/1 -> [Electricals]
  Mux4/1 -> Mux3/1

== system Test_FourMotor_PID_Ave/Detailed/Speed Sensor1 ==
  Ideal Rotational Motion Sensor : fl_lib/Mechanical/Mechanical Sensors/Ideal Rotational Motion Sensor  reference=foundation.enum.MeasurementReference.difference  acceleration_port=false  velocity_port=true  position_port=true  wrap_angle=simscape.enum.onoff.off  offset=0 rad
  Mechanical Rotational Reference : fl_lib/Mechanical/Rotational Elements/Mechanical Rotational Reference
  PS-Simulink Converter : nesl_utility/PS-Simulink Converter  PhysicalDomain=network_engine_domain  SubClassName=ps_output  LeftPortType=input  RightPortType=output  PseudoPeriodic=off  Frequencies=[]  VectorFormat=1-D array  Unit=rpm  AffineConversion=off
  Solver Configuration : nesl_utility/Solver Configuration  PhysicalDomain=network_engine_domain  SubClassName=solver  LeftPortType=input  RightPortType=generic  Tones=[]  Harmonics=[]  SimulateNoise=off  Profile=off  UseLocalSampling=off  EnableSwitchedLinearOptims=on  FrequencyDomain=off  UseCCode=off  RelTol=0.001  AbsTol=0.001  MinStep=1e-09  ToWorkspace=off  RevertToSquareIcSolve=off  NumHomotopyIterations=100  PhasorMode=off  PhasorModeNumHarmonics=1  ConsistencySolver=NEWTON_XTOL_AFTER_FTOL  IndexReductionMethod=DerivativeReplacement  DoDC=off  ResidualTolerance=1e-09  ConsistencyTolSource=GLOBAL  ConsistencyAbsTol=0.001  ConsistencyRelTol=0.001  ConsistencyTolFactor=0.001  UseLocalSolver=off  LocalSolverChoice=NE_BACKWARD_EULER_ADVANCER  ResolveIndetEquations=on  FunctionEvalNumThread=1  LocalSolverSampleTime=0.001  DoFixedCost=off  MaxNonlinIter=3  MaxModeIter=2  ComputeImpulses=off  ImpulseIterations=2  LinearAlgebra=auto  LinearAlgebraNumThread=0  EquationFormulation=NE_TIME_EF  DelaysMemoryBudget=1024  AutomaticFiltering=on  FilteringTimeConstant=0.001  PartitionStorageMethod=AS_NEEDED  PartitionMemoryBudget=1024  PartitionMethod=ROBUST  MultibodyUseLocalSolver=off  MultibodyLocalSolverChoice=ODE1  MultibodyLocalSolverSampleTime=0.001
  Sh : PMIOPort  Side=Left
  Sh1 : PMIOPort  Port=2  Side=Right
  tag scope: Mot_RPM_SYS_1=global
  wires:
  PS-Simulink Converter/1 -> [Mot_RPM_SYS_1]  "Mot_RPM"
  connections:
  Ideal Rotational Motion Sensor/RConn1 -- Mechanical Rotational Reference/LConn1
  Sh1/RConn1 -- Solver Configuration/RConn1 -- Ideal Rotational Motion Sensor/LConn1 -- Sh/RConn1
  PS-Simulink Converter/LConn1 -- Ideal Rotational Motion Sensor/RConn2

== system Test_FourMotor_PID_Ave/Detailed/Speed Sensor2 ==
  Ideal Rotational Motion Sensor : fl_lib/Mechanical/Mechanical Sensors/Ideal Rotational Motion Sensor  reference=foundation.enum.MeasurementReference.difference  acceleration_port=false  velocity_port=true  position_port=true  wrap_angle=simscape.enum.onoff.off  offset=0 rad
  Mechanical Rotational Reference : fl_lib/Mechanical/Rotational Elements/Mechanical Rotational Reference
  PS-Simulink Converter : nesl_utility/PS-Simulink Converter  PhysicalDomain=network_engine_domain  SubClassName=ps_output  LeftPortType=input  RightPortType=output  PseudoPeriodic=off  Frequencies=[]  VectorFormat=1-D array  Unit=rpm  AffineConversion=off
  Solver Configuration : nesl_utility/Solver Configuration  PhysicalDomain=network_engine_domain  SubClassName=solver  LeftPortType=input  RightPortType=generic  Tones=[]  Harmonics=[]  SimulateNoise=off  Profile=off  UseLocalSampling=off  EnableSwitchedLinearOptims=on  FrequencyDomain=off  UseCCode=off  RelTol=0.001  AbsTol=0.001  MinStep=1e-09  ToWorkspace=off  RevertToSquareIcSolve=off  NumHomotopyIterations=100  PhasorMode=off  PhasorModeNumHarmonics=1  ConsistencySolver=NEWTON_XTOL_AFTER_FTOL  IndexReductionMethod=DerivativeReplacement  DoDC=off  ResidualTolerance=1e-09  ConsistencyTolSource=GLOBAL  ConsistencyAbsTol=0.001  ConsistencyRelTol=0.001  ConsistencyTolFactor=0.001  UseLocalSolver=off  LocalSolverChoice=NE_BACKWARD_EULER_ADVANCER  ResolveIndetEquations=on  FunctionEvalNumThread=1  LocalSolverSampleTime=0.001  DoFixedCost=off  MaxNonlinIter=3  MaxModeIter=2  ComputeImpulses=off  ImpulseIterations=2  LinearAlgebra=auto  LinearAlgebraNumThread=0  EquationFormulation=NE_TIME_EF  DelaysMemoryBudget=1024  AutomaticFiltering=on  FilteringTimeConstant=0.001  PartitionStorageMethod=AS_NEEDED  PartitionMemoryBudget=1024  PartitionMethod=ROBUST  MultibodyUseLocalSolver=off  MultibodyLocalSolverChoice=ODE1  MultibodyLocalSolverSampleTime=0.001
  Sh : PMIOPort  Side=Left
  Sh1 : PMIOPort  Port=2  Side=Right
  tag scope: Mot_RPM_SYS_2=global
  wires:
  PS-Simulink Converter/1 -> [Mot_RPM_SYS_2]  "Mot_RPM"
  connections:
  Ideal Rotational Motion Sensor/RConn1 -- Mechanical Rotational Reference/LConn1
  Sh1/RConn1 -- Solver Configuration/RConn1 -- Ideal Rotational Motion Sensor/LConn1 -- Sh/RConn1
  PS-Simulink Converter/LConn1 -- Ideal Rotational Motion Sensor/RConn2

== system Test_FourMotor_PID_Ave/Detailed/Speed Sensor3 ==
  Ideal Rotational Motion Sensor : fl_lib/Mechanical/Mechanical Sensors/Ideal Rotational Motion Sensor  reference=foundation.enum.MeasurementReference.difference  acceleration_port=false  velocity_port=true  position_port=true  wrap_angle=simscape.enum.onoff.off  offset=0 rad
  Mechanical Rotational Reference : fl_lib/Mechanical/Rotational Elements/Mechanical Rotational Reference
  PS-Simulink Converter : nesl_utility/PS-Simulink Converter  PhysicalDomain=network_engine_domain  SubClassName=ps_output  LeftPortType=input  RightPortType=output  PseudoPeriodic=off  Frequencies=[]  VectorFormat=1-D array  Unit=rpm  AffineConversion=off
  Solver Configuration : nesl_utility/Solver Configuration  PhysicalDomain=network_engine_domain  SubClassName=solver  LeftPortType=input  RightPortType=generic  Tones=[]  Harmonics=[]  SimulateNoise=off  Profile=off  UseLocalSampling=off  EnableSwitchedLinearOptims=on  FrequencyDomain=off  UseCCode=off  RelTol=0.001  AbsTol=0.001  MinStep=1e-09  ToWorkspace=off  RevertToSquareIcSolve=off  NumHomotopyIterations=100  PhasorMode=off  PhasorModeNumHarmonics=1  ConsistencySolver=NEWTON_XTOL_AFTER_FTOL  IndexReductionMethod=DerivativeReplacement  DoDC=off  ResidualTolerance=1e-09  ConsistencyTolSource=GLOBAL  ConsistencyAbsTol=0.001  ConsistencyRelTol=0.001  ConsistencyTolFactor=0.001  UseLocalSolver=off  LocalSolverChoice=NE_BACKWARD_EULER_ADVANCER  ResolveIndetEquations=on  FunctionEvalNumThread=1  LocalSolverSampleTime=0.001  DoFixedCost=off  MaxNonlinIter=3  MaxModeIter=2  ComputeImpulses=off  ImpulseIterations=2  LinearAlgebra=auto  LinearAlgebraNumThread=0  EquationFormulation=NE_TIME_EF  DelaysMemoryBudget=1024  AutomaticFiltering=on  FilteringTimeConstant=0.001  PartitionStorageMethod=AS_NEEDED  PartitionMemoryBudget=1024  PartitionMethod=ROBUST  MultibodyUseLocalSolver=off  MultibodyLocalSolverChoice=ODE1  MultibodyLocalSolverSampleTime=0.001
  Sh : PMIOPort  Side=Left
  Sh1 : PMIOPort  Port=2  Side=Right
  tag scope: Mot_RPM_SYS_3=global
  wires:
  PS-Simulink Converter/1 -> [Mot_RPM_SYS_3]  "Mot_RPM"
  connections:
  Ideal Rotational Motion Sensor/RConn1 -- Mechanical Rotational Reference/LConn1
  Sh1/RConn1 -- Solver Configuration/RConn1 -- Ideal Rotational Motion Sensor/LConn1 -- Sh/RConn1
  PS-Simulink Converter/LConn1 -- Ideal Rotational Motion Sensor/RConn2

== system Test_FourMotor_PID_Ave/Detailed/Speed Sensor4 ==
  Ideal Rotational Motion Sensor : fl_lib/Mechanical/Mechanical Sensors/Ideal Rotational Motion Sensor  reference=foundation.enum.MeasurementReference.difference  acceleration_port=false  velocity_port=true  position_port=true  wrap_angle=simscape.enum.onoff.off  offset=0 rad
  Mechanical Rotational Reference : fl_lib/Mechanical/Rotational Elements/Mechanical Rotational Reference
  PS-Simulink Converter : nesl_utility/PS-Simulink Converter  PhysicalDomain=network_engine_domain  SubClassName=ps_output  LeftPortType=input  RightPortType=output  PseudoPeriodic=off  Frequencies=[]  VectorFormat=1-D array  Unit=rpm  AffineConversion=off
  Solver Configuration : nesl_utility/Solver Configuration  PhysicalDomain=network_engine_domain  SubClassName=solver  LeftPortType=input  RightPortType=generic  Tones=[]  Harmonics=[]  SimulateNoise=off  Profile=off  UseLocalSampling=off  EnableSwitchedLinearOptims=on  FrequencyDomain=off  UseCCode=off  RelTol=0.001  AbsTol=0.001  MinStep=1e-09  ToWorkspace=off  RevertToSquareIcSolve=off  NumHomotopyIterations=100  PhasorMode=off  PhasorModeNumHarmonics=1  ConsistencySolver=NEWTON_XTOL_AFTER_FTOL  IndexReductionMethod=DerivativeReplacement  DoDC=off  ResidualTolerance=1e-09  ConsistencyTolSource=GLOBAL  ConsistencyAbsTol=0.001  ConsistencyRelTol=0.001  ConsistencyTolFactor=0.001  UseLocalSolver=off  LocalSolverChoice=NE_BACKWARD_EULER_ADVANCER  ResolveIndetEquations=on  FunctionEvalNumThread=1  LocalSolverSampleTime=0.001  DoFixedCost=off  MaxNonlinIter=3  MaxModeIter=2  ComputeImpulses=off  ImpulseIterations=2  LinearAlgebra=auto  LinearAlgebraNumThread=0  EquationFormulation=NE_TIME_EF  DelaysMemoryBudget=1024  AutomaticFiltering=on  FilteringTimeConstant=0.001  PartitionStorageMethod=AS_NEEDED  PartitionMemoryBudget=1024  PartitionMethod=ROBUST  MultibodyUseLocalSolver=off  MultibodyLocalSolverChoice=ODE1  MultibodyLocalSolverSampleTime=0.001
  Sh : PMIOPort  Side=Left
  Sh1 : PMIOPort  Port=2  Side=Right
  tag scope: Mot_RPM_SYS_4=global
  wires:
  PS-Simulink Converter/1 -> [Mot_RPM_SYS_4]  "Mot_RPM"
  connections:
  Ideal Rotational Motion Sensor/RConn1 -- Mechanical Rotational Reference/LConn1
  Sh1/RConn1 -- Solver Configuration/RConn1 -- Ideal Rotational Motion Sensor/LConn1 -- Sh/RConn1
  PS-Simulink Converter/LConn1 -- Ideal Rotational Motion Sensor/RConn2
